simulink model "hcu_main_ADASwEPS"  (Simulink 8.2)
settings: Solver=FixedStepDiscrete  StartTime=0.0  StopTime=inf  FixedStep=0.001  RelTol=1e-3
PostLoadFcn:
  | , if any(exist('dsrtsu_mdlpostloadfcn', 'file') == [2, 3, 6]), try dsrtsu_mdlpostloadfcn('Execute', bdroot); catch fprintf('Error in PostLoadFcn (dsrtsu_mdlpostloadfcn) for model "%s":\n %s\n', bdroot, lasterr); end, end,
values from neighbouring files (symbols this model uses):
  C_TASK_1MS_S = (	C_TICK_TIME_S       )    [hcu_local_hdr.m]    (also in temp_ovrd_values.m = double(	0.001                  ))
  C_TASK_5MS_S = (	C_TICK_TIME_S      	)    [hcu_local_hdr.m]
  ENUM_ADASLFCSTATUS_OFF = uint8(  0  )    [hcu_local_hdr.m]
  ENUM_ADASLFCSTATUS_STANDBY = uint8(  1  )    [hcu_local_hdr.m]
  ENUM_ADASLKASTATUS_ACTIVE = uint8(  2  )    [hcu_local_hdr.m]
  ENUM_ADASLKASTATUS_OFF = uint8(  0  )    [hcu_local_hdr.m]
  ENUM_ADASLKASTATUS_STANDBY = uint8(  1  )    [hcu_local_hdr.m]
  ENUM_EPSMODEREQ_ANGLE = uint8(  1  )    [hcu_local_hdr.m]
  ENUM_EPSMODEREQ_INTERNAL = uint8(  0  )    [hcu_local_hdr.m]
  ENUM_EPSMODEREQ_TORQUE = uint8(  2  )    [hcu_local_hdr.m]
  ENUM_GEARPOSN_1ST = uint8(  1  )    [hcu_local_hdr.m]
  ENUM_GEARPOSN_2ND = uint8(  2  )    [hcu_local_hdr.m]
  ENUM_GEARPOSN_3RD = uint8(  3  )    [hcu_local_hdr.m]
  ENUM_GEARPOSN_4TH = uint8(  4  )    [hcu_local_hdr.m]
  ENUM_GEARPOSN_5TH = uint8(  5  )    [hcu_local_hdr.m]
  ENUM_GEARPOSN_6TH = uint8(  6  )    [hcu_local_hdr.m]
  ENUM_GEARPOSN_PN = uint8(  0  )    [hcu_local_hdr.m]
  ENUM_GEARPOSN_R = uint8(  7  )    [hcu_local_hdr.m]
  FALSE = boolean( 0 )    [hcu_local_hdr.m]
  TRUE = boolean( 1 )    [hcu_local_hdr.m]
undefined symbols (not defined in the file or in its folder): AACC_DistCtrlIMult_X_mps2, AACC_DistCtrlPMult_X_mps2, AACC_GearActual_enum, AACC_SpdCtrlIMult_X_mps2, AACC_SpdCtrlPMult_X_mps2, AACC_VehSpd_kph, AISP_EPSCurrent_pct, AISP_TqASensorDelta_pct, AISP_TqBSensorDelta_pct, ENUM_ACCSTATUS_ACTIVE, ENUM_ACCSTATUS_OFF, ENUM_ACCSTATUS_STANDBY, ENUM_ADASLFCSTATUS_ACTIVE, ENUM_ADASLFCSTATUS_TRANSITION, ENUM_LFCCCONTSTATUS_ACTIVE, ENUM_LFCCCONTSTATUS_NOTAVAIL_TEMP, ENUM_LFCCCONTSTATUS_OFF, ENUM_LFCCCONTSTATUS_READY, ENUM_LFCCCONTSTATUS_TRANSITION, ENUM_LKACCONTSTATUS_ACTIVE, ENUM_LKACCONTSTATUS_NOTAVAIL_TEMP, ENUM_LKACCONTSTATUS_OFF, ENUM_LKACCONTSTATUS_READY, KACC_AcclReqMax_g, KACC_AcclReqMin_g, KACC_ACCSetTimeGapDef1_s, KACC_ACCSetTimeGapDef2_s, KACC_ACCSetTimeGapDef3_s, KACC_ACCSetTimeGapDef4_s, KACC_ACCSetTimeGapDef5_s, KACC_AirDensity_kgpm3, KACC_AirDragCoef_rat, KACC_CommandsOn_flg, KACC_CruzSpdChgTimeThres_s, KACC_DecReqSwOffThres_Nm, KACC_DecReqSwOnThres_Nm, KACC_DistCtrlAdjTime_s, KACC_DistCtrlCalRate_s, KACC_DistCtrlIC_mps2, KACC_DistCtrlIGain_rat, KACC_DistCtrlIMax_mps2, KACC_DistCtrlIMin_mps2, KACC_DistCtrlIRest_flg, KACC_DistCtrlKGain_rat, KACC_DistCtrlPause_flg, KACC_DistCtrlPGain_rat, KACC_FinalDriveEff_pct, KACC_FinalDriveRatio_rat, KACC_FrontalArea_m2, KACC_GearBoxEff_pct, KACC_LongPushSpdChg_kph, KACC_MaxAccSetSpd_kph, KACC_MinAccSetSpd_kph, KACC_SetAllowSpdLim_kph, KACC_SpdCtrlAdjTime_s, KACC_SpdCtrlCalRate_s, KACC_SpdCtrlIC_mps2, KACC_SpdCtrlIGain_rat, KACC_SpdCtrlIMax_mps2, KACC_SpdCtrlIMin_mps2 ... (+26)
libraries: simulink x54, adas_lib x6, rti1401lib_dio_type3 x4, rtimmsu_dsrtlib x3, hcu_lib x2, aeb x1, ddm x1, dfr x1, dgi x1, dhp x1, dinr x1, dip x1
(part 8 of 9)

== system hcu_main_ADASwEPS/ISP/TqProcessing/TqSensorBZero/Latch ==
  in : Inport
  update : Inport  Port=2
  Delay : Delay  DelayLength=1  InitialCondition=50
  Switch2 : Switch  Criteria=u2 ~= 0  Threshold=0.5
      settings: AttributesFormatString=<Criteria=%<Criteria>>
  out : Outport
  wires:
  update/1 -> Switch2/2
  Switch2/1 -> Delay/1, out/1
  in/1 -> Switch2/1
  Delay/1 -> Switch2/3

== system hcu_main_ADASwEPS/ISP/TqProcessing/TqSensorBZero/Timer ==
  Enable : EnablePort  StatesWhenEnabling=reset
  C_TASK_1MS_S : Constant  Value=C_TASK_1MS_S
  Sum : Sum  Inputs=|++
  Unit Delay : UnitDelay  SampleTime=-1
  Unit Delay1 : UnitDelay  SampleTime=-1
  Time_s : Outport  OutputWhenDisabled=reset  InitialOutput=[0]
  wires:
  C_TASK_1MS_S/1 -> Unit Delay1/1
  Sum/1 -> Unit Delay/1, Time_s/1  "Time_s"
  Unit Delay/1 -> Sum/2
  Unit Delay1/1 -> Sum/1

== system hcu_main_ADASwEPS/OSP/OSP/CheckSum Calculation/Byte0 ==
  BISP_outputs : Inport
  Bus Selector : BusSelector  OutputSignals=VISP_StrAng_deg
  Data Type Conversion : DataTypeConversion  OutDataTypeStr=uint16
  Data Type Conversion1 : DataTypeConversion  OutDataTypeStr=uint16
  Data Type Conversion2 : DataTypeConversion  OutDataTypeStr=uint8
  Data Type Conversion3 : DataTypeConversion  OutDataTypeStr=uint8
  Extract Bits : simulink/Logic and Bit Operations/Extract Bits  bitsToExtract=Upper half  numBits=8  bitIdxRange=[0 7]  outScalingMode=Preserve fixed-point scaling
  Extract Bits1 : simulink/Logic and Bit Operations/Extract Bits  bitsToExtract=Lower half  numBits=8  bitIdxRange=[0 7]  outScalingMode=Preserve fixed-point scaling
  SAS_Angle_cvt : Subsystem  mask(ConvertOut){gain=0.1, offset=-900}
      mask help:
      | Conversion Formula
      |
      | The conversion formula is
      |
      | raw_value = (physical_value - Offset) / Factor
      |
      | where physical_value is the value of the signal after it is saturated using the specified Min and Max values. raw_value is the packed signal value.
  Shift Arithmetic : ArithShift  BitShiftNumber=8
  Byte0 : Outport
  ForByte1 : Outport  Port=2
  wires:
  BISP_outputs/1 -> Bus Selector/1
  Bus Selector/1 -> SAS_Angle_cvt/1(value)  "<VISP_StrAng_deg>"
  SAS_Angle_cvt/1(raw32) -> Data Type Conversion/1
  Data Type Conversion2/1 -> ForByte1/1
  Data Type Conversion1/1 -> Shift Arithmetic/1
  Extract Bits/1 -> Data Type Conversion1/1
  Shift Arithmetic/1 -> Data Type Conversion3/1
  Data Type Conversion3/1 -> Byte0/1
  Extract Bits1/1 -> Data Type Conversion2/1
  Data Type Conversion/1 -> Extract Bits/1, Extract Bits1/1

== system hcu_main_ADASwEPS/OSP/OSP/CheckSum Calculation/Byte1 ==
  ForByte1 : Inport
  Data Type Conversion3 : DataTypeConversion  OutDataTypeStr=uint8
  Byte1 : Outport
  wires:
  Data Type Conversion3/1 -> Byte1/1
  ForByte1/1 -> Data Type Conversion3/1

== system hcu_main_ADASwEPS/OSP/OSP/CheckSum Calculation/Byte2 ==
  Constant1 : Constant  Value=0
  Data Type Conversion3 : DataTypeConversion  OutDataTypeStr=uint8
  Byte2 : Outport
  wires:
  Constant1/1 -> Data Type Conversion3/1
  Data Type Conversion3/1 -> Byte2/1

== system hcu_main_ADASwEPS/OSP/OSP/CheckSum Calculation/Byte3 ==
  BISP_outputs : Inport
  Bus Selector : BusSelector  OutputSignals=VISP_StrAngSensorValid_flg,VISP_StrAngValid_flg
  Data Type Conversion1 : DataTypeConversion  OutDataTypeStr=uint8
  Data Type Conversion2 : DataTypeConversion  OutDataTypeStr=uint8
  Data Type Conversion3 : DataTypeConversion  OutDataTypeStr=uint8
  Sum : Sum  Inputs=2
  bit1 : ArithShift  BitShiftNumber=-1
  Byte3 : Outport
  wires:
  Sum/1 -> Data Type Conversion3/1
  BISP_outputs/1 -> Bus Selector/1
  bit1/1 -> Sum/2
  Data Type Conversion3/1 -> Byte3/1
  Data Type Conversion1/1 -> Sum/1
  Data Type Conversion2/1 -> bit1/1
  Bus Selector/1 -> Data Type Conversion1/1  "<VISP_StrAngSensorValid_flg>"
  Bus Selector/2 -> Data Type Conversion2/1  "<VISP_StrAngValid_flg>"

== system hcu_main_ADASwEPS/OSP/OSP/CheckSum Calculation/ChecksumCalculation ==
  Byte0 : Inport
  Byte1 : Inport  Port=2
  Byte2 : Inport  Port=3
  Byte3 : Inport  Port=4
  SAS_MsgCount : Inport  Port=5
  Bitwise Operator1 : simulink/Logic and Bit Operations/Bitwise Operator  logicop=XOR  UseBitMask=off  NumInputPorts=4  BitMask=bin2dec('11011001')  BitMaskRealWorld=Stored Integer
  Bitwise Operator2 : simulink/Logic and Bit Operations/Bitwise Operator  logicop=XOR  UseBitMask=off  NumInputPorts=3  BitMask=bin2dec('11011001')  BitMaskRealWorld=Stored Integer
  Data Type Conversion{1,3,6..9} (6 alike) : DataTypeConversion  OutDataTypeStr=uint8
  Extract Bits5 : simulink/Logic and Bit Operations/Extract Bits  bitsToExtract=Lower half  numBits=8  bitIdxRange=[0 7]  outScalingMode=Preserve fixed-point scaling
  Extract Bits6 : simulink/Logic and Bit Operations/Extract Bits  bitsToExtract=Upper half  numBits=8  bitIdxRange=[0 7]  outScalingMode=Preserve fixed-point scaling
  Shift Arithmetic2 : ArithShift  BitShiftNumber=4
  Message_Checksum : Outport
  wires:
  Byte1/1 -> Data Type Conversion3/1
  Extract Bits6/1 -> Data Type Conversion7/1
  Extract Bits5/1 -> Data Type Conversion8/1
  Data Type Conversion7/1 -> Shift Arithmetic2/1
  Byte2/1 -> Data Type Conversion6/1
  Byte3/1 -> Data Type Conversion9/1
  Byte0/1 -> Data Type Conversion1/1
  Data Type Conversion1/1 -> Bitwise Operator1/1
  Data Type Conversion3/1 -> Bitwise Operator1/2
  Data Type Conversion6/1 -> Bitwise Operator1/3
  Data Type Conversion9/1 -> Bitwise Operator1/4
  Bitwise Operator1/1 -> Extract Bits6/1, Extract Bits5/1
  Shift Arithmetic2/1 -> Bitwise Operator2/1
  Data Type Conversion8/1 -> Bitwise Operator2/2
  SAS_MsgCount/1 -> Bitwise Operator2/3
  Bitwise Operator2/1 -> Message_Checksum/1

== system hcu_main_ADASwEPS/OSP/OSP/CheckSum Calculation1/Byte0 ==
  Data Type Conversion3 : DataTypeConversion  OutDataTypeStr=uint8
  Elect_PWR_Consumpt : Constant  Value=0
  Elect_PWR_Consumpt_cvt : Subsystem  mask(ConvertOut){gain=0.5, offset=0}
      mask help:
      | Conversion Formula
      |
      | The conversion formula is
      |
      | raw_value = (physical_value - Offset) / Factor
      |
      | where physical_value is the value of the signal after it is saturated using the specified Min and Max values. raw_value is the packed signal value.
  Byte0 : Outport
  wires:
  Elect_PWR_Consumpt/1 -> Elect_PWR_Consumpt_cvt/1(value)
  Data Type Conversion3/1 -> Byte0/1
  Elect_PWR_Consumpt_cvt/1(raw32) -> Data Type Conversion3/1

== system hcu_main_ADASwEPS/OSP/OSP/CheckSum Calculation1/Byte1 ==
  BISP_outputs : Inport
  Bus Selector : BusSelector  OutputSignals=VISP_EPSTqOnShaftValid_flg,VISP_StrAngValid_flg
  Data Type Conversion{1..4} (4 alike) : DataTypeConversion  OutDataTypeStr=uint8
  EpasFailed : Constant  Value=FALSE
  Logical Operator : Logic  Operator=NOT  AllPortsSameDT=off  OutDataTypeStr=boolean
  Sum : Sum  Inputs=3
  bit6 : ArithShift  BitShiftNumber=-6
  bit7 : ArithShift  BitShiftNumber=-7
  Byte1 : Outport
  wires:
  Sum/1 -> Data Type Conversion3/1
  BISP_outputs/1 -> Bus Selector/1
  bit6/1 -> Sum/2
  Data Type Conversion3/1 -> Byte1/1
  Data Type Conversion1/1 -> Sum/1
  Data Type Conversion2/1 -> bit6/1
  Bus Selector/1 -> Logical Operator/1  "<VISP_EPSTqOnShaftValid_flg>"
  Bus Selector/2 -> Data Type Conversion2/1  "<VISP_StrAngValid_flg>"
  Logical Operator/1 -> Data Type Conversion1/1
  Data Type Conversion4/1 -> bit7/1
  EpasFailed/1 -> Data Type Conversion4/1
  bit7/1 -> Sum/3

== system hcu_main_ADASwEPS/OSP/OSP/CheckSum Calculation1/Byte2 ==
  BISP_outputs : Inport
  Bus Selector : BusSelector  OutputSignals=VISP_EPSTqOnShaft_Nm
  Data Type Conversion3 : DataTypeConversion  OutDataTypeStr=uint8
  Steering_Torque_cvt : Subsystem  mask(ConvertOut){gain=0.1794, offset=-22.78}
      mask help:
      | Conversion Formula
      |
      | The conversion formula is
      |
      | raw_value = (physical_value - Offset) / Factor
      |
      | where physical_value is the value of the signal after it is saturated using the specified Min and Max values. raw_value is the packed signal value.
  Byte2 : Outport
  wires:
  Steering_Torque_cvt/1(raw32) -> Data Type Conversion3/1
  Data Type Conversion3/1 -> Byte2/1
  Bus Selector/1 -> Steering_Torque_cvt/1(value)  "<VISP_EPSTqOnShaft_Nm>"
  BISP_outputs/1 -> Bus Selector/1

== system hcu_main_ADASwEPS/OSP/OSP/CheckSum Calculation1/Byte3 ==
  BISP_outputs : Inport
  Bus Selector : BusSelector  OutputSignals=VISP_RelStrAng_deg
  Data Type Conversion : DataTypeConversion  OutDataTypeStr=uint16
  Data Type Conversion1 : DataTypeConversion  OutDataTypeStr=uint16
  Data Type Conversion2 : DataTypeConversion  OutDataTypeStr=uint8
  Data Type Conversion3 : DataTypeConversion  OutDataTypeStr=uint8
  Extract Bits : simulink/Logic and Bit Operations/Extract Bits  bitsToExtract=Upper half  numBits=8  bitIdxRange=[0 7]  outScalingMode=Preserve fixed-point scaling
  Extract Bits1 : simulink/Logic and Bit Operations/Extract Bits  bitsToExtract=Lower half  numBits=8  bitIdxRange=[0 7]  outScalingMode=Preserve fixed-point scaling
  R_SAS_Angle_cvt : Subsystem  mask(ConvertOut){gain=0.1, offset=-1400}
      mask help:
      | Conversion Formula
      |
      | The conversion formula is
      |
      | raw_value = (physical_value - Offset) / Factor
      |
      | where physical_value is the value of the signal after it is saturated using the specified Min and Max values. raw_value is the packed signal value.
  Shift Arithmetic : ArithShift  BitShiftNumber=8
  Byte3 : Outport
  ForByte4 : Outport  Port=2
  wires:
  BISP_outputs/1 -> Bus Selector/1
  Bus Selector/1 -> R_SAS_Angle_cvt/1(value)  "<VISP_RelStrAng_deg>"
  R_SAS_Angle_cvt/1(raw32) -> Data Type Conversion/1
  Data Type Conversion2/1 -> ForByte4/1
  Data Type Conversion1/1 -> Shift Arithmetic/1
  Extract Bits/1 -> Data Type Conversion1/1
  Shift Arithmetic/1 -> Data Type Conversion3/1
  Data Type Conversion3/1 -> Byte3/1
  Extract Bits1/1 -> Data Type Conversion2/1
  Data Type Conversion/1 -> Extract Bits/1, Extract Bits1/1

== system hcu_main_ADASwEPS/OSP/OSP/CheckSum Calculation1/ChecksumCalculation ==
  Byte0 : Inport
  Byte1 : Inport  Port=2
  Byte2 : Inport  Port=3
  Byte3 : Inport  Port=4
  EPAS2_MsgCount : Inport  Port=5
  Bitwise Operator1 : simulink/Logic and Bit Operations/Bitwise Operator  logicop=XOR  UseBitMask=off  NumInputPorts=4  BitMask=bin2dec('11011001')  BitMaskRealWorld=Stored Integer
  Bitwise Operator2 : simulink/Logic and Bit Operations/Bitwise Operator  logicop=XOR  UseBitMask=off  NumInputPorts=3  BitMask=bin2dec('11011001')  BitMaskRealWorld=Stored Integer
  Data Type Conversion{1,3,6..9} (6 alike) : DataTypeConversion  OutDataTypeStr=uint8
  Extract Bits5 : simulink/Logic and Bit Operations/Extract Bits  bitsToExtract=Lower half  numBits=8  bitIdxRange=[0 7]  outScalingMode=Preserve fixed-point scaling
  Extract Bits6 : simulink/Logic and Bit Operations/Extract Bits  bitsToExtract=Upper half  numBits=8  bitIdxRange=[0 7]  outScalingMode=Preserve fixed-point scaling
  Shift Arithmetic2 : ArithShift  BitShiftNumber=4
  Message_Checksum : Outport
  wires:
  Bitwise Operator2/1 -> Message_Checksum/1
  EPAS2_MsgCount/1 -> Bitwise Operator2/3
  Data Type Conversion8/1 -> Bitwise Operator2/2
  Shift Arithmetic2/1 -> Bitwise Operator2/1
  Bitwise Operator1/1 -> Extract Bits5/1, Extract Bits6/1
  Data Type Conversion9/1 -> Bitwise Operator1/4
  Data Type Conversion6/1 -> Bitwise Operator1/3
  Data Type Conversion3/1 -> Bitwise Operator1/2
  Data Type Conversion1/1 -> Bitwise Operator1/1
  Byte0/1 -> Data Type Conversion1/1
  Byte3/1 -> Data Type Conversion9/1
  Byte2/1 -> Data Type Conversion6/1
  Data Type Conversion7/1 -> Shift Arithmetic2/1
  Extract Bits5/1 -> Data Type Conversion8/1
  Extract Bits6/1 -> Data Type Conversion7/1
  Byte1/1 -> Data Type Conversion3/1

== system hcu_main_ADASwEPS/RTI Data/RTI Data Store/RTI Data Store/RTI Data Store ==
  RTI Data Store : Subsystem  mask(RTI_DATA_STORE){}
      mask help:
      | RTI Data Store Block. This block is used by RTI to store internal model dependent data. Deleting this block will result in data loss.
      |
      | NEVER DELETE, COPY, OR MODIFY THIS BLOCK!
      mask Help:
      | RTI Data Store Block. This block is used by RTI to store internal model dependent data. Deleting this block will result in data loss.
      | 
      | NEVER DELETE, COPY, OR MODIFY THIS BLOCK!
      mask Display: text(0.5, 0.5, ' ', 'HorizontalAlignment', 'center');

== system hcu_main_ADASwEPS/APPH/ACC/ACC/ACCStatus_SetSpeed_SetTimeGap/InForwardGear ==
  VDINR_NowGearPosn_enum : Inport
  Constant : Constant  Value=ENUM_GEARPOSN_1ST
  Constant1 : Constant  Value=ENUM_GEARPOSN_2ND
  Constant2 : Constant  Value=ENUM_GEARPOSN_3RD
  Constant3 : Constant  Value=ENUM_GEARPOSN_4TH
  Constant4 : Constant  Value=ENUM_GEARPOSN_5TH
  Constant5 : Constant  Value=ENUM_GEARPOSN_6TH
  Logical Operator : Logic  Operator=OR  Inputs=6  AllPortsSameDT=off  OutDataTypeStr=boolean
  Relational Operator{,1..5} (6 alike) : RelationalOperator  Operator===  OutDataTypeStr=boolean
  VACC_InForwardGear_flg : Outport
  wires:
  Logical Operator/1 -> VACC_InForwardGear_flg/1  "VACC_InForwardGear_flg"
  Constant/1 -> Relational Operator/2
  Constant1/1 -> Relational Operator1/2
  Constant2/1 -> Relational Operator2/2
  Constant3/1 -> Relational Operator3/2
  Constant4/1 -> Relational Operator4/2
  VDINR_NowGearPosn_enum/1 -> Relational Operator5/1, Relational Operator4/1, Relational Operator3/1, Relational Operator2/1, Relational Operator1/1, Relational Operator/1
  Constant5/1 -> Relational Operator5/2
  Relational Operator/1 -> Logical Operator/1
  Relational Operator1/1 -> Logical Operator/2
  Relational Operator2/1 -> Logical Operator/3
  Relational Operator3/1 -> Logical Operator/4
  Relational Operator4/1 -> Logical Operator/5
  Relational Operator5/1 -> Logical Operator/6

== system hcu_main_ADASwEPS/APPH/ACC/ACC/ACCStatus_SetSpeed_SetTimeGap/InPNGear ==
  VDINR_NowGearPosn_enum : Inport
  Constant : Constant  Value=ENUM_GEARPOSN_PN
  Relational Operator : RelationalOperator  Operator===  OutDataTypeStr=boolean
  VACC_InPNGear_flg : Outport
  wires:
  VDINR_NowGearPosn_enum/1 -> Relational Operator/1
  Constant/1 -> Relational Operator/2
  Relational Operator/1 -> VACC_InPNGear_flg/1  "VACC_InPNGear_flg"

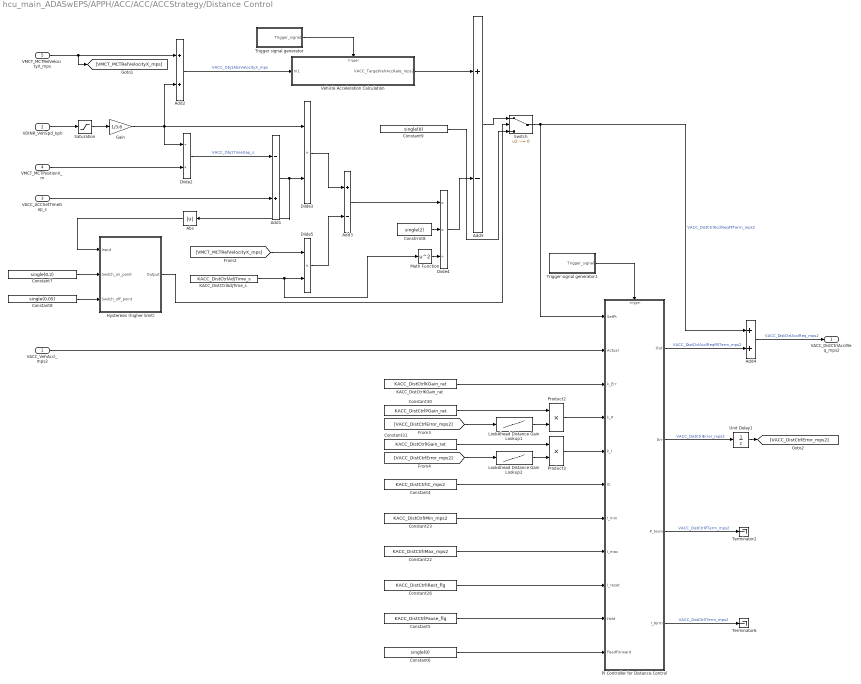
== system hcu_main_ADASwEPS/APPH/ACC/ACC/ACCStrategy/Distance Control ==
  VACC_VehAccl_mps2 : Inport
  VDINR_VehSpd_kph : Inport  Port=2
  VACC_ACCSetTimeGap_s : Inport  Port=3
  VMCT_MCTPositionX_m : Inport  Port=4
  VMCT_MCTRelVelocityX_mps : Inport  Port=5
  Abs : Abs
  Add1 : Sum  Inputs=-+
  Add2 : Sum
  Add3 : Sum  Inputs=+-
  Add4 : Sum
  Add5 : Sum  Inputs=+-
  Constant22 : Constant  Value=KACC_DistCtrlIMax_mps2
  Constant23 : Constant  Value=KACC_DistCtrlIMin_mps2
  Constant26 : Constant  Value=KACC_DistCtrlIRest_flg
  Constant30 : Constant  Value=KACC_DistCtrlPGain_rat
  Constant31 : Constant  Value=KACC_DistCtrlIGain_rat
  Constant4 : Constant  Value=KACC_DistCtrlIC_mps2
  Constant5 : Constant  Value=KACC_DistCtrlPause_flg
  Constant6 : Constant  Value=single(0)
  Constant7 : Constant  Value=single(0.2)
  Constant8 : Constant  Value=single(0.05)
  Constant9 : Constant  Value=single(0)
  Constrrnt8 : Constant  Value=single(2)
  Diide2 : Product  Inputs=/*
  Diide3 : Product  Inputs=**
  Diide4 : Product  Inputs=**/
  Diide5 : Product  Inputs=**
  Gain : Gain  Gain=1/3.6
  Hysteresis (higher limit) : Subsystem  TreatAsAtomicUnit=on
  KACC_DistCtrlAdjTime_s : Constant  Value=KACC_DistCtrlAdjTime_s
  KACC_DistCtrlKGain_rat : Constant  Value=KACC_DistCtrlKGain_rat
  LookAhead Distance Gain Lookup1 : Lookup  InputValues=AACC_DistCtrlPMult_X_mps2  Table=MACC_DistCtrlPMult_rat  LookUpMeth=Interpolation-Use End Values
      settings: AttributesFormatString=%<InputValues>\n%<Table>
  LookAhead Distance Gain Lookup2 : Lookup  InputValues=AACC_DistCtrlIMult_X_mps2  Table=MACC_DistCtrlIMult_rat  LookUpMeth=Interpolation-Use End Values
      settings: AttributesFormatString=%<InputValues>\n%<Table>
  Math Function : Math  Operator=square  SaturateOnIntegerOverflow=on
  PI Controller for Distance Control : Subsystem  TreatAsAtomicUnit=on
  Product2 : Product  OutDataTypeStr=single  RndMeth=Zero
  Product3 : Product  OutDataTypeStr=single  RndMeth=Zero
  Saturation : Saturate  UpperLimit=inf  LowerLimit=20
  Switch : Switch  Criteria=u2 ~= 0
  Terminator2 : Terminator
  Terminator6 : Terminator
  Trigger signal generator : Subsystem  TreatAsAtomicUnit=on
  Trigger signal generator1 : Subsystem  TreatAsAtomicUnit=on
  Unit Delay1 : UnitDelay  SampleTime=-1
  Vehicle Acceleration Calculation : Subsystem
  VACC_DistCtrlAcclReq_mps2 : Outport
  wires:
  Add1/1 -> Abs/1, Diide3/2
  Diide3/1 -> Add3/1
  Diide5/1 -> Add3/2
  Add3/1 -> Diide4/1
  Math Function/1 -> Diide4/3
  Constrrnt8/1 -> Diide4/2
  Diide4/1 -> Add5/2
  VDINR_VehSpd_kph/1 -> Saturation/1
  KACC_DistCtrlAdjTime_s/1 -> Math Function/1, Diide5/2
  Gain/1 -> Add2/2, Diide2/1, Diide3/1
  VMCT_MCTPositionX_m/1 -> Diide2/2
  VACC_ACCSetTimeGap_s/1 -> Add1/2
  Diide2/1 -> Add1/1  "VACC_Obj1TimeGap_s"
  [VMCT_MCTRelVelocityX_mps] -> Diide5/1
  VMCT_MCTRelVelocityX_mps/1 -> Add2/1, [VMCT_MCTRelVelocityX_mps]
  Add2/1 -> Vehicle Acceleration Calculation/1(In1)  "VACC_Obj1AbsVelocityX_mps"
  Trigger signal generator/1(Trigger_signal) -> Vehicle Acceleration Calculation/Trigger
  Vehicle Acceleration Calculation/1(VACC_TargetVehAccRate_mps2) -> Add5/1
  KACC_DistCtrlKGain_rat/1 -> PI Controller for Distance Control/3(k_Err)
  Product3/1 -> PI Controller for Distance Control/5(k_I)
  Product2/1 -> PI Controller for Distance Control/4(k_P)
  Constant30/1 -> Product2/1
  LookAhead Distance Gain Lookup1/1 -> Product2/2
  [VACC_DistCtrlError_mps2] -> LookAhead Distance Gain Lookup1/1
  LookAhead Distance Gain Lookup2/1 -> Product3/2
  Constant31/1 -> Product3/1
  [VACC_DistCtrlError_mps2] -> LookAhead Distance Gain Lookup2/1
  Unit Delay1/1 -> [VACC_DistCtrlError_mps2]
  PI Controller for Distance Control/2(Err) -> Unit Delay1/1  "VACC_DistCtrlError_mps2"
  Constant23/1 -> PI Controller for Distance Control/7(I_min)
  Constant22/1 -> PI Controller for Distance Control/8(I_max)
  Constant26/1 -> PI Controller for Distance Control/9(I_reset)
  Constant4/1 -> PI Controller for Distance Control/6(IC)
  PI Controller for Distance Control/3(P_term) -> Terminator2/1  "VACC_DistCtrlPTerm_mps2"
  PI Controller for Distance Control/4(I_term) -> Terminator6/1  "VACC_DistCtrlITerm_mps2"
  PI Controller for Distance Control/1(Out) -> Add4/2  "VACC_DistCtrlAcclReqFBTerm_mps2"
  Add4/1 -> VACC_DistCtrlAcclReq_mps2/1  "VACC_DistCtrlAcclReq_mps2"
  Switch/1 -> PI Controller for Distance Control/1(SetPt), Add4/1  "VACC_DistCtrlAcclReqFFTerm_mps2"
  Trigger signal generator1/1(Trigger_signal) -> PI Controller for Distance Control/Trigger
  VACC_VehAccl_mps2/1 -> PI Controller for Distance Control/2(Actual)
  Constant5/1 -> PI Controller for Distance Control/10(Hold)
  Constant6/1 -> PI Controller for Distance Control/11(FeedForward)
  Constant7/1 -> Hysteresis (higher limit)/2(Switch_on_point)
  Constant8/1 -> Hysteresis (higher limit)/3(Switch_off_point)
  Hysteresis (higher limit)/1(Output) -> Switch/2
  Add5/1 -> Switch/1
  Constant9/1 -> Switch/3
  Abs/1 -> Hysteresis (higher limit)/1(Input)
  Saturation/1 -> Gain/1

== system hcu_main_ADASwEPS/APPH/ACC/ACC/ACCStrategy/Speed Control ==
  VACC_ACCSetSpd_kph : Inport
  VDINR_VehSpd_kph : Inport  Port=2
  VACC_VehAccl_mps2 : Inport  Port=3
  Add : Sum  Inputs=+-
  Add1 : Sum
  Constant22 : Constant  Value=KACC_SpdCtrlIMax_mps2
  Constant23 : Constant  Value=KACC_SpdCtrlIMin_mps2
  Constant26 : Constant  Value=KACC_SpdCtrlIRest_flg
  Constant3 : Constant  Value=KACC_SpdCtrlIC_mps2
  Constant30 : Constant  Value=KACC_SpdCtrlPGain_rat
  Constant31 : Constant  Value=KACC_SpdCtrlIGain_rat
  Constant4 : Constant  Value=KACC_SpdCtrlPause_flg
  Constant5 : Constant  Value=single(0)
  Diide : Product  Inputs=*/
  Gain : Gain  Gain=1/3.6
  Gain1 : Gain  Gain=1/3.6
  KACC_SpdCtrlAdjTime_s : Constant  Value=KACC_SpdCtrlAdjTime_s
  KACC_SpdCtrlKGain_rat : Constant  Value=KACC_SpdCtrlKGain_rat
  LookAhead Distance Gain Lookup1 : Lookup  InputValues=AACC_SpdCtrlPMult_X_mps2  Table=MACC_SpdCtrlPMult_rat  LookUpMeth=Interpolation-Use End Values
      settings: AttributesFormatString=%<InputValues>\n%<Table>
  LookAhead Distance Gain Lookup2 : Lookup  InputValues=AACC_SpdCtrlIMult_X_mps2  Table=MACC_SpdCtrlIMult_rat  LookUpMeth=Interpolation-Use End Values
      settings: AttributesFormatString=%<InputValues>\n%<Table>
  PI Controller for Seepd Control : Subsystem  TreatAsAtomicUnit=on
  Product2 : Product  OutDataTypeStr=single  RndMeth=Zero
  Product3 : Product  OutDataTypeStr=single  RndMeth=Zero
  Terminator2 : Terminator
  Terminator6 : Terminator
  Trigger signal generator : Subsystem  TreatAsAtomicUnit=on
  Unit Delay1 : UnitDelay  SampleTime=-1
  VACC_SpdCtrlAcclReq_mps2 : Outport
  wires:
  Diide/1 -> PI Controller for Seepd Control/1(SetPt), Add1/1  "VACC_SpdCtrlAcclReqFFTerm_mps2"
  KACC_SpdCtrlAdjTime_s/1 -> Diide/2
  Add/1 -> Diide/1
  VDINR_VehSpd_kph/1 -> Gain1/1
  VACC_ACCSetSpd_kph/1 -> Gain/1
  KACC_SpdCtrlKGain_rat/1 -> PI Controller for Seepd Control/3(k_Err)
  Product3/1 -> PI Controller for Seepd Control/5(k_I)
  Product2/1 -> PI Controller for Seepd Control/4(k_P)
  Constant30/1 -> Product2/1
  LookAhead Distance Gain Lookup1/1 -> Product2/2
  [VACC_SpdCtrlError_mps2] -> LookAhead Distance Gain Lookup1/1
  LookAhead Distance Gain Lookup2/1 -> Product3/2
  Constant31/1 -> Product3/1
  [VACC_SpdCtrlError_mps2] -> LookAhead Distance Gain Lookup2/1
  Unit Delay1/1 -> [VACC_SpdCtrlError_mps2]
  PI Controller for Seepd Control/2(Err) -> Unit Delay1/1  "VACC_SpdCtrlError_mps2"
  Constant23/1 -> PI Controller for Seepd Control/7(I_min)
  Constant22/1 -> PI Controller for Seepd Control/8(I_max)
  Constant26/1 -> PI Controller for Seepd Control/9(I_reset)
  Constant3/1 -> PI Controller for Seepd Control/6(IC)
  PI Controller for Seepd Control/3(P_term) -> Terminator2/1  "VACC_SpdCtrlPTerm_mps2"
  PI Controller for Seepd Control/4(I_term) -> Terminator6/1  "VACC_SpdCtrlITerm_mps2"
  PI Controller for Seepd Control/1(Out) -> Add1/2  "VACC_SpdCtrlAcclReqFBTerm_mps2"
  Add1/1 -> VACC_SpdCtrlAcclReq_mps2/1  "VACC_SpdCtrlAcclReq_mps2"
  Trigger signal generator/1(Trigger_signal) -> PI Controller for Seepd Control/Trigger
  Gain/1 -> Add/1
  VACC_VehAccl_mps2/1 -> PI Controller for Seepd Control/2(Actual)
  Constant4/1 -> PI Controller for Seepd Control/10(Hold)
  Constant5/1 -> PI Controller for Seepd Control/11(FeedForward)
  Gain1/1 -> Add/2

== system hcu_main_ADASwEPS/APPH/ACC/ACC/ACCStrategy/Timer ==
  Enable : EnablePort  StatesWhenEnabling=reset
  C_TASK_5MS_S : Constant  Value=C_TASK_5MS_S
  Sum : Sum  Inputs=|++
  Unit Delay : UnitDelay  SampleTime=-1
  Unit Delay1 : UnitDelay  SampleTime=-1
  SineTime_s : Outport  OutputWhenDisabled=reset  InitialOutput=[0]
  wires:
  Unit Delay1/1 -> Sum/1
  Unit Delay/1 -> Sum/2
  Sum/1 -> SineTime_s/1, Unit Delay/1  "SineTime_s"
  C_TASK_5MS_S/1 -> Unit Delay1/1

== system hcu_main_ADASwEPS/APPH/ACC/ACC/ACCStrategy/Torque Estimation ==
  VACC_AcclReqFinal_mps2 : Inport
  VDINR_VehSpd_kph : Inport  Port=2
  VDINR_NowGearPosn_enum : Inport  Port=3
  VDINR_EngSpd_rpm : Inport  Port=4
  Add2 : Sum  Inputs=+++
  Constant : Constant  Value=KACC_VehicleMass_kg
  Constant1 : Constant  Value=KACC_AirDensity_kgpm3
  Constant2 : Constant  Value=KACC_AirDragCoef_rat
  Constant3 : Constant  Value=KACC_FrontalArea_m2
  Constant4 : Constant  Value=single(0.5)
  Diide1 : Product  Inputs=*****
  Diide5 : Product  Inputs=**
  FinalDrive : Subsystem
  Gain : Gain  Gain=1/3.6
  Gain1 : Gain  Gain=9.8
  GearRatio : Subsystem
  LookAhead Distance Gain Lookup1 : Lookup  InputValues=AACC_VehSpd_kph  Table=MACC_TireRollResistance_Nm  LookUpMeth=Interpolation-Use End Values
      settings: AttributesFormatString=%<InputValues>\n%<Table>
  Math Function : Math  Operator=square  SaturateOnIntegerOverflow=on
  Tire : Subsystem
  TqConverter : Subsystem
  VACC_TqReqRaw_Nm : Outport
  wires:
  Constant/1 -> Diide5/2
  Diide5/1 -> Add2/1
  VACC_AcclReqFinal_mps2/1 -> Diide5/1
  Constant4/1 -> Diide1/2
  Diide1/1 -> Add2/2
  VDINR_VehSpd_kph/1 -> Math Function/1, Gain/1, Tire/2(VehSpd)
  Math Function/1 -> Diide1/1
  Tire/1(TqOut_tire) -> FinalDrive/1(TqIn_FD)
  Tire/2(OmegaOut_tire) -> FinalDrive/2(OmegaIn_FD)
  FinalDrive/1(TqOut_FD) -> GearRatio/1(TqIn_GB)
  FinalDrive/2(OmegaOut_FD) -> GearRatio/2(OmegaIn_GB)
  GearRatio/1(TqOut_GB) -> TqConverter/1(TqIn_TC)
  GearRatio/2(OmegaOut_GB) -> TqConverter/2(OmegaIn_TC)
  TqConverter/1(VACC_TqReqRaw_Nm) -> VACC_TqReqRaw_Nm/1
  Add2/1 -> Tire/1(Fx)
  Constant1/1 -> Diide1/3
  Constant3/1 -> Diide1/5
  Constant2/1 -> Diide1/4
  VDINR_NowGearPosn_enum/1 -> GearRatio/3(GearActual)
  VDINR_EngSpd_rpm/1 -> TqConverter/3(VDINR_EngSpd_rpm)
  Gain/1 -> LookAhead Distance Gain Lookup1/1
  LookAhead Distance Gain Lookup1/1 -> Gain1/1
  Gain1/1 -> Add2/3

== system hcu_main_ADASwEPS/APPH/ACC/ACC/ACCStrategy/Trigger signal generator ==
  Constant3 : Constant  Value=KACC_VehAccCalRate_s
  trigger signal generator : Subsystem  TreatAsAtomicUnit=on
  Trigger_signal : Outport
  wires:
  trigger signal generator/1(Trigger_signal) -> Trigger_signal/1
  Constant3/1 -> trigger signal generator/1(Time_dur [s])

== system hcu_main_ADASwEPS/APPH/ACC/ACC/ACCStrategy/Vehicle Acceleration Calculation ==
  note: m/s^2
  note: m/s
  note: km/h
  In1 : Inport
  Trigger : TriggerPort
  Constant1 : Constant  Value=KACC_VehAccCalRate_s
  Constant2 : Constant  Value=KACC_VehAccCalRate_s
  Constant3 : Constant  Value=KACC_VehAccCalRate_s
  Constant4 : Constant  Value=KACC_VehAccFltConst_s
  Divide : Product  Inputs=*/
  Divide1 : Product  Inputs=*/
  Gain : Gain  Gain=1000/3600
  Gain1 : Gain  Gain=1/9.81  OutDataTypeStr=single
  Sum : Sum  Inputs=+-
  Sum1 : Sum  Inputs=+-
  Terminator : Terminator
  Terminator1 : Terminator
  Unit Delay : UnitDelay  SampleTime=-1
  Unit Delay1 : UnitDelay  SampleTime=-1
  signal_filter : Subsystem
  VACC_VehAccl_mps2 : Outport
  wires:
  Gain1/1 -> Terminator1/1  "VACC_VehAccl_g"
  Divide1/1 -> Terminator/1  "VACC_VehJerk_mps3"
  Constant1/1 -> Divide1/2
  Sum1/1 -> Divide1/1
  Unit Delay1/1 -> Sum1/2
  signal_filter/1(raw_input_filt) -> Gain1/1, VACC_VehAccl_mps2/1, Unit Delay1/1, Sum1/1  "VACC_VehAccl_mps2"
  Constant3/1 -> Divide/2
  Gain/1 -> Divide/1
  Sum/1 -> Gain/1
  Unit Delay/1 -> Sum/2
  In1/1 -> Sum/1, Unit Delay/1
  Constant2/1 -> signal_filter/3(Ts)
  Constant4/1 -> signal_filter/2(Tc)
  Divide/1 -> signal_filter/1(raw_input)  "VACC_VehAcclUnFlt_mps2"

== system hcu_main_ADASwEPS/APPH/ACC/ACC/CommandDetermination/Hysteresis (higher limit) ==
  Input : Inport
  Switch_on_point : Inport  Port=2
  Switch_off_point : Inport  Port=3
  Data Type Conversion : DataTypeConversion
  Logical Operator1 : Logic  AllPortsSameDT=off  OutDataTypeStr=boolean
  Logical Operator2 : Logic  Operator=NOT  AllPortsSameDT=off  OutDataTypeStr=boolean
  Logical Operator3 : Logic  Operator=OR  AllPortsSameDT=off  OutDataTypeStr=boolean
  Relational Operator : RelationalOperator  OutDataTypeStr=boolean
  Relational Operator1 : RelationalOperator  Operator=<=  OutDataTypeStr=boolean
  Unit Delay : UnitDelay  SampleTime=-1
  Output : Outport
  wires:
  Switch_on_point/1 -> Relational Operator/2
  Switch_off_point/1 -> Relational Operator1/2
  Logical Operator2/1 -> Logical Operator1/2
  Logical Operator1/1 -> Unit Delay/1, Data Type Conversion/1
  Unit Delay/1 -> Logical Operator3/1
  Input/1 -> Relational Operator/1, Relational Operator1/1
  Relational Operator/1 -> Logical Operator3/2
  Logical Operator3/1 -> Logical Operator1/1
  Relational Operator1/1 -> Logical Operator2/1
  Data Type Conversion/1 -> Output/1

== system hcu_main_ADASwEPS/APPH/ACC/ACC/CommandDetermination/Hysteresis (lower limit) ==
  Input : Inport
  Switch_on_point : Inport  Port=2
  Switch_off_point : Inport  Port=3
  Data Type Conversion : DataTypeConversion
  Logical Operator1 : Logic  AllPortsSameDT=off  OutDataTypeStr=boolean
  Logical Operator2 : Logic  Operator=NOT  AllPortsSameDT=off  OutDataTypeStr=boolean
  Logical Operator3 : Logic  Operator=OR  AllPortsSameDT=off  OutDataTypeStr=boolean
  Relational Operator : RelationalOperator  Operator=<=  OutDataTypeStr=boolean
  Relational Operator1 : RelationalOperator  OutDataTypeStr=boolean
  Unit Delay : UnitDelay  SampleTime=-1
  Output : Outport
  wires:
  Switch_on_point/1 -> Relational Operator/2
  Switch_off_point/1 -> Relational Operator1/2
  Logical Operator2/1 -> Logical Operator1/2
  Logical Operator1/1 -> Unit Delay/1, Data Type Conversion/1
  Unit Delay/1 -> Logical Operator3/1
  Input/1 -> Relational Operator/1, Relational Operator1/1
  Relational Operator/1 -> Logical Operator3/2
  Logical Operator3/1 -> Logical Operator1/1
  Relational Operator1/1 -> Logical Operator2/1
  Data Type Conversion/1 -> Output/1

== system hcu_main_ADASwEPS/EPSS/EPSS/AngleMode/Angle2Torque/Hysteresis (higher limit) ==
  Input : Inport
  Switch_on_point : Inport  Port=2
  Switch_off_point : Inport  Port=3
  Data Type Conversion : DataTypeConversion
  Logical Operator1 : Logic  AllPortsSameDT=off  OutDataTypeStr=boolean
  Logical Operator2 : Logic  Operator=NOT  AllPortsSameDT=off  OutDataTypeStr=boolean
  Logical Operator3 : Logic  Operator=OR  AllPortsSameDT=off  OutDataTypeStr=boolean
  Relational Operator : RelationalOperator  OutDataTypeStr=boolean
  Relational Operator1 : RelationalOperator  Operator=<=  OutDataTypeStr=boolean
  Unit Delay : UnitDelay  SampleTime=-1
  Output : Outport
  wires:
  Switch_on_point/1 -> Relational Operator/2
  Switch_off_point/1 -> Relational Operator1/2
  Logical Operator2/1 -> Logical Operator1/2
  Logical Operator1/1 -> Unit Delay/1, Data Type Conversion/1
  Unit Delay/1 -> Logical Operator3/1
  Input/1 -> Relational Operator/1, Relational Operator1/1
  Relational Operator/1 -> Logical Operator3/2
  Logical Operator3/1 -> Logical Operator1/1
  Relational Operator1/1 -> Logical Operator2/1
  Data Type Conversion/1 -> Output/1

== system hcu_main_ADASwEPS/EPSS/EPSS/AngleMode/Angle2Torque/InverseAssistTable ==
  VEPSS_MotPWMReqAngle_pct : Inport
  VDINR_VehSpd_kph : Inport  Port=2
  MEPSS_EPSMotPWMRescalingInv_pct : Lookup  InputValues=[-250 -3 0 3 250]  Table=[-100 -3 0 3 100]  LookUpMeth=Interpolation-Use End Values
      settings: AttributesFormatString="Input=\"%<InputValues>\"\\nOutput=\"%<Table>\""
  MEPSS_TqAssistPWM_pct : Lookup  InputValues=[-20 -19 -18 -17 -16 -15 -14 -13 -12 -11 -10 -9 -8 -7 -6 -5 -4 -3 -2 -1 0 1 2 3 4 5 6 7 8 9 10 11 12 13 14 15 16 17 18 19 20]  Table=[-10:0.5:10]  LookUpMeth=Interpolation-Use End Values
      settings: AttributesFormatString="Input=\"%<InputValues>\"\\nOutput=\"%<Table>\""
  MEPSS_VehSpdPWMMult_rat : Lookup  InputValues=[-100 -80 -60 -40 -20 -10 0 10 20 40 60 80 100]  Table=[1 1 1 1 1 1 1 1 1 1 1 1 1]  LookUpMeth=Interpolation-Use End Values
      settings: AttributesFormatString="Input=\"%<InputValues>\"\\nOutput=\"%<Table>\""
  Product : Product  Inputs=*/
  VEPSS_StrWhlTqReqAngRaw_Nm : Outport
  wires:
  MEPSS_EPSMotPWMRescalingInv_pct/1 -> Product/1
  VEPSS_MotPWMReqAngle_pct/1 -> MEPSS_EPSMotPWMRescalingInv_pct/1
  VDINR_VehSpd_kph/1 -> MEPSS_VehSpdPWMMult_rat/1
  MEPSS_VehSpdPWMMult_rat/1 -> Product/2
  Product/1 -> MEPSS_TqAssistPWM_pct/1
  MEPSS_TqAssistPWM_pct/1 -> VEPSS_StrWhlTqReqAngRaw_Nm/1  "VEPSS_StrWhlTqReqAngRaw_Nm"

== system hcu_main_ADASwEPS/EPSS/EPSS/AngleMode/Angle2Torque/Rate_Limit ==
  Data_Input : Inport
  Rising_Rate : Inport  Port=2
  Falling_Rate : Inport  Port=3
  Initial_condition : Inport  Port=4
  Enable : EnablePort  StatesWhenEnabling=reset
  RateLimiter : Subsystem
  Data_Output : Outport  OutputWhenDisabled=reset  InitialOutput=[0]
  wires:
  RateLimiter/1(Data_Output) -> Data_Output/1
  Data_Input/1 -> RateLimiter/1(Data_Input)
  Initial_condition/1 -> RateLimiter/4(Initial_Condition)
  Falling_Rate/1 -> RateLimiter/3(Falling Rate)
  Rising_Rate/1 -> RateLimiter/2(Rising Rate)

== system hcu_main_ADASwEPS/EPSS/EPSS/EPSTest/SignalPlayer/Timer ==
  Enable : EnablePort  StatesWhenEnabling=reset
  C_TASK_1MS_S : Constant  Value=C_TASK_1MS_S
  Sum : Sum  Inputs=|++
  Unit Delay : UnitDelay  SampleTime=-1
  Unit Delay1 : UnitDelay  SampleTime=-1
  SineTime_s : Outport  OutputWhenDisabled=reset  InitialOutput=[0]
  wires:
  Unit Delay1/1 -> Sum/1
  Unit Delay/1 -> Sum/2
  Sum/1 -> SineTime_s/1, Unit Delay/1  "SineTime_s"
  C_TASK_1MS_S/1 -> Unit Delay1/1

== system hcu_main_ADASwEPS/EPSS/EPSS/EPSTest/SignalPlayer/Timer1 ==
  Enable : EnablePort  StatesWhenEnabling=reset
  C_TASK_1MS_S : Constant  Value=C_TASK_1MS_S
  Sum : Sum  Inputs=|++
  Unit Delay : UnitDelay  SampleTime=-1
  Unit Delay1 : UnitDelay  SampleTime=-1
  SineTime_s : Outport  OutputWhenDisabled=reset  InitialOutput=[0]
  wires:
  C_TASK_1MS_S/1 -> Unit Delay1/1
  Sum/1 -> Unit Delay/1, SineTime_s/1  "SineTime_s"
  Unit Delay/1 -> Sum/2
  Unit Delay1/1 -> Sum/1

== system hcu_main_ADASwEPS/OSP/OSP/CheckSum Calculation/Byte0/SAS_Angle_cvt ==
  value : Inport
  Add : Sum  Inputs=+-
  Data Type Conversion : DataTypeConversion  OutDataTypeStr=uint32  RndMeth=Nearest
  Divide : Product  Inputs=*/
  gain : Constant  Value=single(gain)  OutDataTypeStr=single
  offset : Constant  Value=single(offset)  OutDataTypeStr=single
  raw32 : Outport
  wires:
  Data Type Conversion/1 -> raw32/1
  gain/1 -> Divide/2
  Add/1 -> Divide/1
  Divide/1 -> Data Type Conversion/1
  offset/1 -> Add/2
  value/1 -> Add/1

== system hcu_main_ADASwEPS/OSP/OSP/CheckSum Calculation1/Byte0/Elect_PWR_Consumpt_cvt ==
  value : Inport
  Add : Sum  Inputs=+-
  Data Type Conversion : DataTypeConversion  OutDataTypeStr=uint32  RndMeth=Nearest
  Divide : Product  Inputs=*/
  gain : Constant  Value=single(gain)  OutDataTypeStr=single
  offset : Constant  Value=single(offset)  OutDataTypeStr=single
  raw32 : Outport
  wires:
  value/1 -> Add/1
  offset/1 -> Add/2
  Divide/1 -> Data Type Conversion/1
  Add/1 -> Divide/1
  gain/1 -> Divide/2
  Data Type Conversion/1 -> raw32/1

== system hcu_main_ADASwEPS/OSP/OSP/CheckSum Calculation1/Byte2/Steering_Torque_cvt ==
  value : Inport
  Add : Sum  Inputs=+-
  Data Type Conversion : DataTypeConversion  OutDataTypeStr=uint32  RndMeth=Nearest
  Divide : Product  Inputs=*/
  gain : Constant  Value=single(gain)  OutDataTypeStr=single
  offset : Constant  Value=single(offset)  OutDataTypeStr=single
  raw32 : Outport
  wires:
  Data Type Conversion/1 -> raw32/1
  gain/1 -> Divide/2
  Add/1 -> Divide/1
  Divide/1 -> Data Type Conversion/1
  offset/1 -> Add/2
  value/1 -> Add/1

== system hcu_main_ADASwEPS/OSP/OSP/CheckSum Calculation1/Byte3/R_SAS_Angle_cvt ==
  value : Inport
  Add : Sum  Inputs=+-
  Data Type Conversion : DataTypeConversion  OutDataTypeStr=uint32  RndMeth=Nearest
  Divide : Product  Inputs=*/
  gain : Constant  Value=single(gain)  OutDataTypeStr=single
  offset : Constant  Value=single(offset)  OutDataTypeStr=single
  raw32 : Outport
  wires:
  Data Type Conversion/1 -> raw32/1
  gain/1 -> Divide/2
  Add/1 -> Divide/1
  Divide/1 -> Data Type Conversion/1
  offset/1 -> Add/2
  value/1 -> Add/1

== system hcu_main_ADASwEPS/RTI Data/RTI Data Store/RTI Data Store/RTI Data Store/RTI Data Store ==

== system hcu_main_ADASwEPS/APPH/ACC/ACC/ACCStrategy/Distance Control/Hysteresis (higher limit) ==
  Input : Inport
  Switch_on_point : Inport  Port=2
  Switch_off_point : Inport  Port=3
  Data Type Conversion : DataTypeConversion
  Logical Operator1 : Logic  AllPortsSameDT=off  OutDataTypeStr=boolean
  Logical Operator2 : Logic  Operator=NOT  AllPortsSameDT=off  OutDataTypeStr=boolean
  Logical Operator3 : Logic  Operator=OR  AllPortsSameDT=off  OutDataTypeStr=boolean
  Relational Operator : RelationalOperator  OutDataTypeStr=boolean
  Relational Operator1 : RelationalOperator  Operator=<=  OutDataTypeStr=boolean
  Unit Delay : UnitDelay  SampleTime=-1
  Output : Outport
  wires:
  Switch_on_point/1 -> Relational Operator/2
  Switch_off_point/1 -> Relational Operator1/2
  Logical Operator2/1 -> Logical Operator1/2
  Logical Operator1/1 -> Unit Delay/1, Data Type Conversion/1
  Unit Delay/1 -> Logical Operator3/1
  Input/1 -> Relational Operator/1, Relational Operator1/1
  Relational Operator/1 -> Logical Operator3/2
  Logical Operator3/1 -> Logical Operator1/1
  Relational Operator1/1 -> Logical Operator2/1
  Data Type Conversion/1 -> Output/1

== system hcu_main_ADASwEPS/APPH/ACC/ACC/ACCStrategy/Distance Control/PI Controller for Distance Control ==
  note: Universal PI Controller
  SetPt : Inport
  Actual : Inport  Port=2
  k_Err : Inport  Port=3
  k_P : Inport  Port=4
  k_I : Inport  Port=5
  IC : Inport  Port=6
  I_min : Inport  Port=7
  I_max : Inport  Port=8
  I_reset : Inport  Port=9
  Hold : Inport  Port=10
  FeedForward : Inport  Port=11
  Trigger : TriggerPort
  Constant : Constant  Value=false  OutDataTypeStr=boolean
  Constant14 : Constant  Value=0  OutDataTypeStr=single
  Data Type Conversion : DataTypeConversion  OutDataTypeStr=single  SaturateOnIntegerOverflow=on  RndMeth=Zero
  Integrator : Subsystem  TreatAsAtomicUnit=on
  Logical Operator : Logic  Operator=OR  AllPortsSameDT=off  OutDataTypeStr=boolean
  Product1 : Product  InputSameDT=on  OutDataTypeStr=Inherit: Same as first input
  Product2 : Product  InputSameDT=on  OutDataTypeStr=Inherit: Same as first input
  Product3 : Product  InputSameDT=on  OutDataTypeStr=Inherit: Same as first input
  Sum : Sum  Inputs=+|+  SaturateOnIntegerOverflow=on  InputSameDT=on  OutDataTypeStr=Inherit: Same as first input
  Sum1 : Sum  Inputs=++|
  Sum2 : Sum  Inputs=+|-  SaturateOnIntegerOverflow=on  InputSameDT=on  OutDataTypeStr=Inherit: Same as first input
  Switch2 : Switch  Criteria=u2 ~= 0
  Switch4 : Switch  Criteria=u2 ~= 0
  Unit Delay : UnitDelay  InitialCondition=true  SampleTime=-1
  Unit Delay1 : UnitDelay  SampleTime=-1
  Out : Outport  OutputWhenDisabled=reset  InitialOutput=[0]
  Err : Outport  Port=2  OutputWhenDisabled=reset  InitialOutput=[0]
  P_term : Outport  Port=3  OutputWhenDisabled=reset  InitialOutput=[0]
  I_term : Outport  Port=4  OutputWhenDisabled=reset  InitialOutput=[0]
  wires:
  Product2/1 -> P_term/1, Sum/1
  Integrator/1(Out) -> I_term/1, Sum/2
  Sum/1 -> Sum1/2
  [HoldReq] -> Switch2/2
  Switch2/1 -> Out/1, Unit Delay1/1
  Unit Delay1/1 -> Switch2/1
  Sum1/1 -> Switch2/3
  FeedForward/1 -> Sum1/1
  Constant14/1 -> Switch4/1
  [HoldReq] -> Switch4/2
  Data Type Conversion/1 -> Switch4/3
  Switch4/1 -> Product3/1, Err/1
  Hold/1 -> [HoldReq]
  Constant/1 -> Unit Delay/1
  Unit Delay/1 -> Logical Operator/1
  I_reset/1 -> Logical Operator/2
  Logical Operator/1 -> Integrator/2(Rst)
  Sum2/1 -> Data Type Conversion/1
  Product3/1 -> Product1/1, Product2/2
  IC/1 -> Integrator/3(IC)
  Product1/1 -> Integrator/1(In)
  k_I/1 -> Product1/2
  k_P/1 -> Product2/1
  k_Err/1 -> Product3/2
  I_min/1 -> Integrator/4(Min)
  I_max/1 -> Integrator/5(Max)
  Actual/1 -> Sum2/2
  SetPt/1 -> Sum2/1

== system hcu_main_ADASwEPS/APPH/ACC/ACC/ACCStrategy/Distance Control/Trigger signal generator ==
  Constant3 : Constant  Value=KACC_TargetVehAccCalRate_s
  trigger signal generator : Subsystem  TreatAsAtomicUnit=on
  Trigger_signal : Outport
  wires:
  trigger signal generator/1(Trigger_signal) -> Trigger_signal/1
  Constant3/1 -> trigger signal generator/1(Time_dur [s])

== system hcu_main_ADASwEPS/APPH/ACC/ACC/ACCStrategy/Distance Control/Trigger signal generator1 ==
  Constant3 : Constant  Value=KACC_DistCtrlCalRate_s
  trigger signal generator : Subsystem  TreatAsAtomicUnit=on
  Trigger_signal : Outport
  wires:
  trigger signal generator/1(Trigger_signal) -> Trigger_signal/1
  Constant3/1 -> trigger signal generator/1(Time_dur [s])

== system hcu_main_ADASwEPS/APPH/ACC/ACC/ACCStrategy/Distance Control/Vehicle Acceleration Calculation ==
  note: m/s^2
  note: m/s
  note: km/h
  In1 : Inport
  Trigger : TriggerPort
  Constant1 : Constant  Value=KACC_TargetVehAccCalRate_s
  Constant2 : Constant  Value=KACC_TargetVehAccCalRate_s
  Constant3 : Constant  Value=KACC_TargetVehAccCalRate_s
  Constant4 : Constant  Value=KACC_TargetVehAccFltConst_s
  Divide : Product  Inputs=*/
  Divide1 : Product  Inputs=*/
  Gain : Gain  Gain=1000/3600
  Gain1 : Gain  Gain=1/9.81  OutDataTypeStr=single
  Gain2 : Gain  Gain=0  OutDataTypeStr=single
  Sum : Sum  Inputs=+-
  Sum1 : Sum  Inputs=+-
  Terminator : Terminator
  Terminator1 : Terminator
  Unit Delay : UnitDelay  SampleTime=-1
  Unit Delay1 : UnitDelay  SampleTime=-1
  signal_filter : Subsystem
  VACC_TargetVehAccRate_mps2 : Outport
  wires:
  Gain1/1 -> Terminator1/1  "VACC_TargetVehAccRate_g"
  Divide1/1 -> Terminator/1  "VACC_TargetVehJerk_mps3"
  Constant1/1 -> Divide1/2
  Sum1/1 -> Divide1/1
  Unit Delay1/1 -> Sum1/2
  signal_filter/1(raw_input_filt) -> Gain2/1  "VACC_TargetVehAccRate_mps2"
  Constant3/1 -> Divide/2
  Gain/1 -> Divide/1
  Sum/1 -> Gain/1
  Unit Delay/1 -> Sum/2
  In1/1 -> Sum/1, Unit Delay/1
  Constant2/1 -> signal_filter/3(Ts)
  Constant4/1 -> signal_filter/2(Tc)
  Divide/1 -> signal_filter/1(raw_input)  "VACC_TargetVehAccRateUnFlt_mps2"
  Gain2/1 -> Gain1/1, VACC_TargetVehAccRate_mps2/1, Unit Delay1/1, Sum1/1

== system hcu_main_ADASwEPS/APPH/ACC/ACC/ACCStrategy/Speed Control/PI Controller for Seepd Control ==
  note: Universal PI Controller
  SetPt : Inport
  Actual : Inport  Port=2
  k_Err : Inport  Port=3
  k_P : Inport  Port=4
  k_I : Inport  Port=5
  IC : Inport  Port=6
  I_min : Inport  Port=7
  I_max : Inport  Port=8
  I_reset : Inport  Port=9
  Hold : Inport  Port=10
  FeedForward : Inport  Port=11
  Trigger : TriggerPort
  Constant : Constant  Value=false  OutDataTypeStr=boolean
  Constant14 : Constant  Value=0  OutDataTypeStr=single
  Data Type Conversion : DataTypeConversion  OutDataTypeStr=single  SaturateOnIntegerOverflow=on  RndMeth=Zero
  Integrator : Subsystem  TreatAsAtomicUnit=on
  Logical Operator : Logic  Operator=OR  AllPortsSameDT=off  OutDataTypeStr=boolean
  Product1 : Product  InputSameDT=on  OutDataTypeStr=Inherit: Same as first input
  Product2 : Product  InputSameDT=on  OutDataTypeStr=Inherit: Same as first input
  Product3 : Product  InputSameDT=on  OutDataTypeStr=Inherit: Same as first input
  Sum : Sum  Inputs=+|+  SaturateOnIntegerOverflow=on  InputSameDT=on  OutDataTypeStr=Inherit: Same as first input
  Sum1 : Sum  Inputs=++|
  Sum2 : Sum  Inputs=+|-  SaturateOnIntegerOverflow=on  InputSameDT=on  OutDataTypeStr=Inherit: Same as first input
  Switch2 : Switch  Criteria=u2 ~= 0
  Switch4 : Switch  Criteria=u2 ~= 0
  Unit Delay : UnitDelay  InitialCondition=true  SampleTime=-1
  Unit Delay1 : UnitDelay  SampleTime=-1
  Out : Outport  OutputWhenDisabled=reset  InitialOutput=[0]
  Err : Outport  Port=2  OutputWhenDisabled=reset  InitialOutput=[0]
  P_term : Outport  Port=3  OutputWhenDisabled=reset  InitialOutput=[0]
  I_term : Outport  Port=4  OutputWhenDisabled=reset  InitialOutput=[0]
  wires:
  Product2/1 -> P_term/1, Sum/1
  Integrator/1(Out) -> I_term/1, Sum/2
  Sum/1 -> Sum1/2
  [HoldReq] -> Switch2/2
  Switch2/1 -> Out/1, Unit Delay1/1
  Unit Delay1/1 -> Switch2/1
  Sum1/1 -> Switch2/3
  FeedForward/1 -> Sum1/1
  Constant14/1 -> Switch4/1
  [HoldReq] -> Switch4/2
  Data Type Conversion/1 -> Switch4/3
  Switch4/1 -> Product3/1, Err/1
  Hold/1 -> [HoldReq]
  Constant/1 -> Unit Delay/1
  Unit Delay/1 -> Logical Operator/1
  I_reset/1 -> Logical Operator/2
  Logical Operator/1 -> Integrator/2(Rst)
  Sum2/1 -> Data Type Conversion/1
  Product3/1 -> Product1/1, Product2/2
  IC/1 -> Integrator/3(IC)
  Product1/1 -> Integrator/1(In)
  k_I/1 -> Product1/2
  k_P/1 -> Product2/1
  k_Err/1 -> Product3/2
  I_min/1 -> Integrator/4(Min)
  I_max/1 -> Integrator/5(Max)
  Actual/1 -> Sum2/2
  SetPt/1 -> Sum2/1

== system hcu_main_ADASwEPS/APPH/ACC/ACC/ACCStrategy/Speed Control/Trigger signal generator ==
  Constant3 : Constant  Value=KACC_SpdCtrlCalRate_s
  trigger signal generator : Subsystem  TreatAsAtomicUnit=on
  Trigger_signal : Outport
  wires:
  trigger signal generator/1(Trigger_signal) -> Trigger_signal/1
  Constant3/1 -> trigger signal generator/1(Time_dur [s])

== system hcu_main_ADASwEPS/APPH/ACC/ACC/ACCStrategy/Torque Estimation/FinalDrive ==
  TqIn_FD : Inport
  OmegaIn_FD : Inport  Port=2
  Constant1 : Constant  Value=KACC_FinalDriveRatio_rat
  Constant2 : Constant  Value=KACC_FinalDriveEff_pct
  Gain : Gain  Gain=1/100
  Product : Product  Inputs=*//  RndMeth=Zero
  Product2 : Product  RndMeth=Zero
  TqOut_FD : Outport
  OmegaOut_FD : Outport  Port=2
  wires:
  Product/1 -> TqOut_FD/1
  TqIn_FD/1 -> Product/1
  Constant1/1 -> Product2/1, Product/3
  OmegaIn_FD/1 -> Product2/2
  Product2/1 -> OmegaOut_FD/1
  Constant2/1 -> Gain/1
  Gain/1 -> Product/2

== system hcu_main_ADASwEPS/APPH/ACC/ACC/ACCStrategy/Torque Estimation/GearRatio ==
  TqIn_GB : Inport
  OmegaIn_GB : Inport  Port=2
  GearActual : Inport  Port=3
  Constant2 : Constant  Value=KACC_GearBoxEff_pct
  Gain : Gain  Gain=1/100
  LookAhead Distance Gain Lookup1 : Lookup  InputValues=AACC_GearActual_enum  Table=MACC_GearRatio_rat  LookUpMeth=Interpolation-Use End Values
      settings: AttributesFormatString=%<InputValues>\n%<Table>
  Product2 : Product  RndMeth=Zero
  Produt3 : Product  Inputs=*//  RndMeth=Zero
  TqOut_GB : Outport
  OmegaOut_GB : Outport  Port=2
  wires:
  Constant2/1 -> Gain/1
  Product2/1 -> OmegaOut_GB/1
  OmegaIn_GB/1 -> Product2/2
  LookAhead Distance Gain Lookup1/1 -> Produt3/3, Product2/1
  TqIn_GB/1 -> Produt3/1
  Produt3/1 -> TqOut_GB/1
  GearActual/1 -> LookAhead Distance Gain Lookup1/1
  Gain/1 -> Produt3/2

== system hcu_main_ADASwEPS/APPH/ACC/ACC/ACCStrategy/Torque Estimation/Tire ==
  Fx : Inport
  VehSpd : Inport  Port=2
  Ad1 : Sum
  Constant : Constant  Value=single(0.1)
  Constant1 : Constant  Value=KACC_TireRadius_m
  Constant2 : Constant  Value=KACC_TireRadius_m
  Constant3 : Constant  Value=KACC_TireRotationalInertia_kgpm2
  Derivative : Subsystem
  Proct2 : Product  RndMeth=Zero
  Product1 : Product  RndMeth=Zero
  Product3 : Product  Inputs=*/  RndMeth=Zero
  trigger signal generator : Subsystem  TreatAsAtomicUnit=on
  TqOut_tire : Outport
  OmegaOut_tire : Outport  Port=2
  wires:
  Constant1/1 -> Product1/2
  Product1/1 -> Ad1/1
  Proct2/1 -> Ad1/2
  Fx/1 -> Product1/1
  Ad1/1 -> TqOut_tire/1
  VehSpd/1 -> Product3/1
  Constant2/1 -> Product3/2
  Product3/1 -> OmegaOut_tire/1, Derivative/2(Omega_tire)  "Omega_tire"
  Derivative/1(AlphaOut_tire) -> Proct2/2
  trigger signal generator/1(Trigger_signal) -> Derivative/Trigger
  Constant/1 -> trigger signal generator/1(Time_dur [s]), Derivative/1(SampleTime)
  Constant3/1 -> Proct2/1
